simulink model "DSM2_2018a"  (R2018a)
settings: Solver=VariableStepAuto  StartTime=0.0  StopTime=0.6  RelTol=1e-3
settings Model: Creator=bzhan  LastModifiedBy=bzhan
settings DataIOCC: ReturnWorkspaceOutputs=on
settings SFSimCC: SimUseLocalCustomCode=on
settings RTWCC: RTWUseLocalCustomCode=on

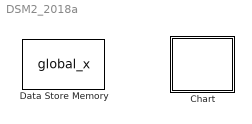
== system DSM2_2018a ==
  Chart : Stateflow chart  TreatAsAtomicUnit=on
  Data Store Memory : DataStoreMemory  DataStoreName=global_x  ReadBeforeWriteMsg=warning  WriteAfterWriteMsg=warning  WriteAfterReadMsg=warning  ShowAdditionalParam=off  OutDataTypeStr=int32

== stateflow chart DSM2_2018a/Chart ==
  settings: updateMethod=DISCRETE  sampleTime=0.1
  state A
  state B
  (default) -> A : {v=global_x;}
  A -> B : {v=v+1;global_x=v;f()}
  B -> A : {v=v+2;global_x=v;f()}
  data: global_x data_store_memory; v local
  function f:
    | function f
    |   fprintf("%d\n", global_x);
